simulink subsystem "potControl"  (R2022b)
settings: Solver=VariableStepAuto  StartTime=0.0  StopTime=10.0  RelTol=1e-3
libraries: pot_test x1, Raptor_lib x1
settings Model: Creator=serga  LastModifiedBy=serga

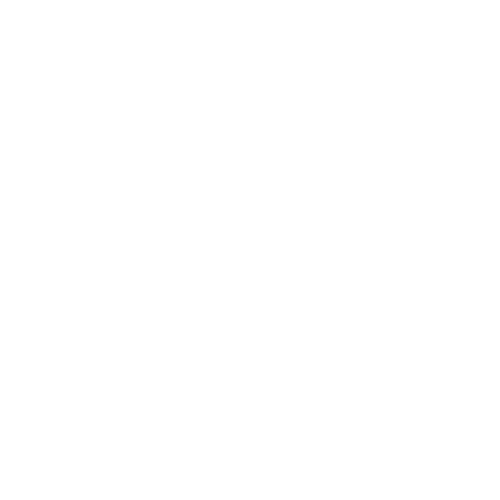
[thumbnail: Simulink's stored preview of the top-level diagram]
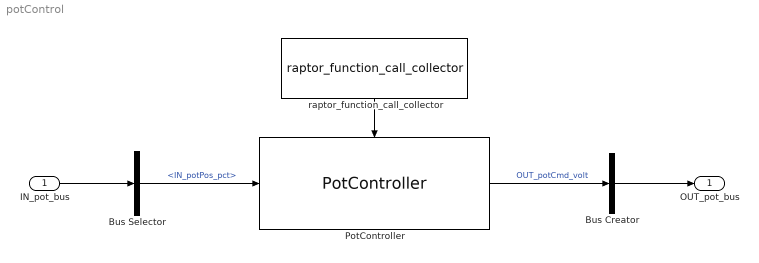
== system potControl ==
  IN_pot_bus : Inport
  Bus Creator : BusCreator  Inputs=1
  Bus Selector : BusSelector  OutputSignals=IN_potPos_pct
  PotController : pot_test/PotController  SystemSampleTime=-1  VariantActivationTime=update diagram  Latency=0  AutoFrameSizeCalculation=off
  raptor_function_call_collector : Raptor_lib/Triggers/raptor_function_call_collector  count=5
      settings: SourceProductName=Raptor
  OUT_pot_bus : Outport
  wires:
  IN_pot_bus/1 -> Bus Selector/1
  Bus Selector/1 -> PotController/1  "<IN_potPos_pct>"
  PotController/1 -> Bus Creator/1  "OUT_potCmd_volt"
  Bus Creator/1 -> OUT_pot_bus/1
  raptor_function_call_collector/1 -> PotController/Trigger
